simulink model "test"  (R2025a)
settings: Solver=VariableStepAuto  StartTime=0.0  StopTime=20  RelTol=1e-3
libraries: simulink_extras x2, aerolibanim x1, aerolibasang x1
settings Model: Creator=Ranvir  LastModifiedBy=Ranvir

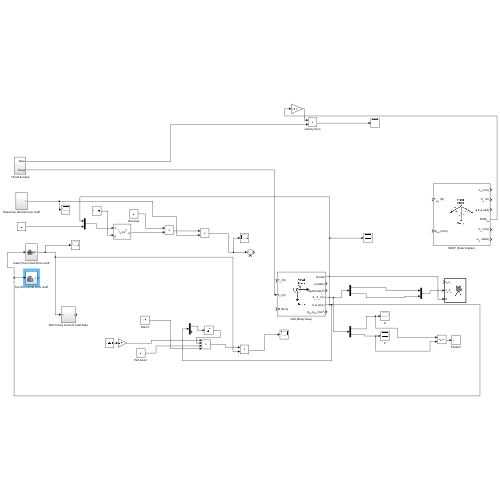
[thumbnail: Simulink's stored preview of the top-level diagram]
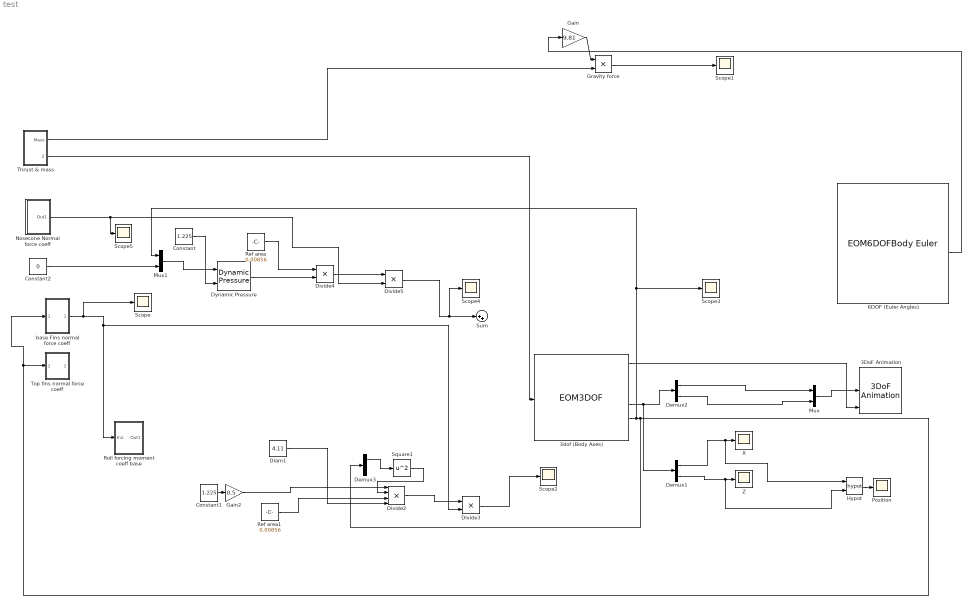
== system test ==
  3DoF Animation : aerolibanim/3DoF Animation  u1=[-25000 10000 -8000 2000 -15050 -3050]  u2=0.05  u3=1.0  u5=Fly alongside  u6=[1000 1000 1000]  u7=2  u8=on
  3dof (Body Axes) : EOM3DOF  v_ini=0  mass=36  Iyy=15
  6DOF (Euler Angles) : EOM6DOFBodyEuler  mass_0=36.51
  Constant : Constant  Value=1.225
  Constant1 : Constant  Value=1.225
  Constant2 : Constant  Value=0
  Demux1 : Demux  Outputs=2
  Demux2 : Demux  Outputs=2
  Demux3 : Demux  Outputs=2
  Diam1 : Constant  Value=4.11
  Divide2 : Product  Inputs=****
  Divide3 : Product  Inputs=**
  Divide4 : Product  Inputs=**
  Divide5 : Product  Inputs=**
  Dynamic Pressure : aerolibasang/Dynamic Pressure
  Gain : Gain  Gain=9.81
  Gain2 : Gain  Gain=0.5
  Gravity force : Product  Inputs=**
  Hypot : Math  Operator=hypot
  Mux : Mux  Inputs=2
  Mux1 : Mux  Inputs=2
  Nosecone Normal force coeff : Subsystem
  Position : Scope
      settings: ActiveDisplayYMinimum=-5509.2409156817193  ActiveDisplayYMaximum=105656.42411552551  DataLoggingVariableName=ScopeData7
  Ref area : Constant  Value=0.00856
  Ref area1 : Constant  Value=0.00856
  Roll forcing moment coeff base : Subsystem
  Scope{,1..5} (6 alike) : Scope
      Scope settings: ActiveDisplayYMinimum=9.6012949698591061  ActiveDisplayYMaximum=9.6019679428376143
      Scope1 settings: ActiveDisplayYMinimum=-90.814917446809943  ActiveDisplayYMaximum=480.58128367549506
      Scope2 settings: ActiveDisplayYMinimum=90.598933136696871  ActiveDisplayYMaximum=96.338960936146933  DataLoggingVariableName=ScopeData4
      Scope3 settings: ActiveDisplayYMinimum=318368.50157545973  ActiveDisplayYMaximum=399063.90685158595  DataLoggingVariableName=ScopeData5
      Scope4 settings: ActiveDisplayYMinimum=-1  ActiveDisplayYMaximum=1  DataLoggingVariableName=ScopeData8
      Scope5 settings: ActiveDisplayYMinimum=0.23621080058183891  ActiveDisplayYMaximum=0.2364376394256005  DataLoggingVariableName=ScopeData9
  Square1 : Math  Operator=square
  Sum : Sum  Inputs=|++
  Thrust & mass : Subsystem
  Top fins normal force coeff : Subsystem
  X : Scope
      settings: ActiveDisplayYMinimum=-6442.9252668406516  ActiveDisplayYMaximum=23566.686005062387  DataLoggingVariableName=ScopeData2
  Z : Scope
      settings: ActiveDisplayYMinimum=-39401.199186369508  ActiveDisplayYMaximum=178036.276331874  DataLoggingVariableName=ScopeData3
  base Fins normal force coeff : Subsystem
  wires:
  Divide5/1 -> Sum/1, Scope4/1
  Diam1/1 -> Divide2/4
  Square1/1 -> Divide2/2
  Divide4/1 -> Divide5/1
  Constant/1 -> Dynamic Pressure/2
  Mux1/1 -> Dynamic Pressure/1
  Divide2/1 -> Divide3/1
  Ref area1/1 -> Divide2/3
  Hypot/1 -> Position/1
  Demux2/1 -> Mux/1
  Demux2/2 -> Mux/2
  Demux1/1 -> Hypot/1, X/1
  Demux1/2 -> Hypot/2, Z/1
  Constant2/1 -> Mux1/2
  3dof (Body Axes)/1 -> 3DoF Animation/3
  Divide3/1 -> Scope2/1
  Dynamic Pressure/1 -> Divide4/2
  Nosecone Normal force coeff/1(Out1) -> Scope5/1, Divide5/2
  Ref area/1 -> Divide4/1
  Constant1/1 -> Gain2/1
  Thrust & mass/2(Thrust) -> 3dof (Body Axes)/2
  Mux/1 -> 3DoF Animation/2
  3dof (Body Axes)/4 -> Demux2/1, Demux1/1
  Demux3/1 -> Square1/1
  6DOF (Euler Angles)/4 -> Gain/1
  3dof (Body Axes)/5 -> base Fins normal force coeff/1(Velocity), Top fins normal force coeff/1(In1), Demux3/1, Scope3/1, Mux1/1
  Gain2/1 -> Divide2/1
  Thrust & mass/1(Mass) -> Gravity force/2
  Gravity force/1 -> Scope1/1
  base Fins normal force coeff/1(Out1) -> Scope/1, Divide3/2, Roll forcing moment coeff base/1(In1)
  Gain/1 -> Gravity force/1

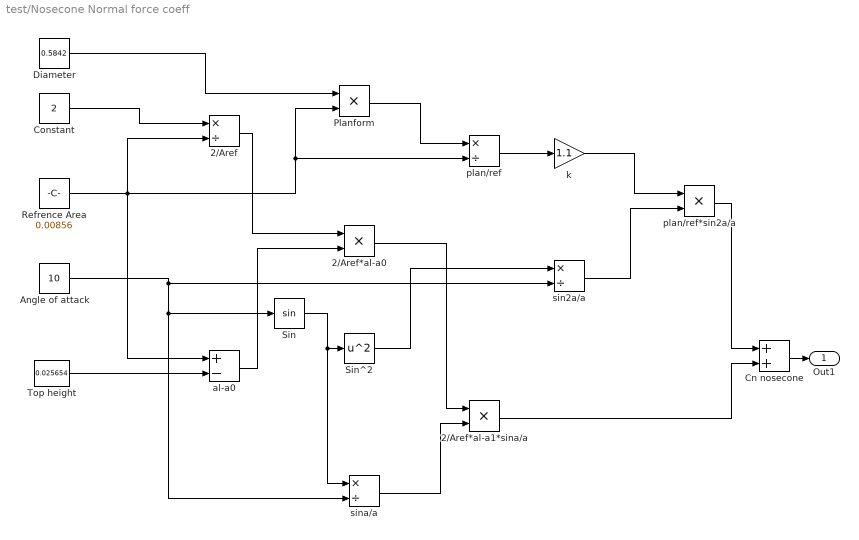
== system test/Nosecone Normal force coeff ==
  2/Aref : Product  Inputs=*/
  2/Aref*al-a0 : Product  Inputs=**
  2/Aref*al-a1*sina/a : Product  Inputs=**
  Angle of attack : Constant  Value=10
  Cn nosecone : Sum
  Constant : Constant  Value=2
  Diameter : Constant  Value=0.5842
  Planform : Product  Inputs=**
  Refrence Area : Constant  Value=0.00856
  Sin : Trigonometry
  Sin^2 : Math  Operator=square
  Top height : Constant  Value=0.025654
  al-a0 : Sum  Inputs=+-
  k : Gain  Gain=1.1
  plan/ref : Product  Inputs=*/
  plan/ref*sin2a/a : Product  Inputs=**
  sin2a/a : Product  Inputs=*/
  sina/a : Product  Inputs=*/
  Out1 : Outport
  wires:
  k/1 -> plan/ref*sin2a/a/1
  Refrence Area/1 -> plan/ref/2, Planform/2, 2/Aref/2, al-a0/1
  Sin^2/1 -> sin2a/a/1
  plan/ref/1 -> k/1
  Angle of attack/1 -> sin2a/a/2, Sin/1, sina/a/2
  al-a0/1 -> 2/Aref*al-a0/2
  2/Aref*al-a0/1 -> 2/Aref*al-a1*sina/a/1
  Sin/1 -> Sin^2/1, sina/a/1
  Diameter/1 -> Planform/1
  2/Aref/1 -> 2/Aref*al-a0/1
  Top height/1 -> al-a0/2
  sina/a/1 -> 2/Aref*al-a1*sina/a/2
  Constant/1 -> 2/Aref/1
  plan/ref*sin2a/a/1 -> Cn nosecone/1
  2/Aref*al-a1*sina/a/1 -> Cn nosecone/2
  Planform/1 -> plan/ref/1
  sin2a/a/1 -> plan/ref*sin2a/a/2
  Cn nosecone/1 -> Out1/1

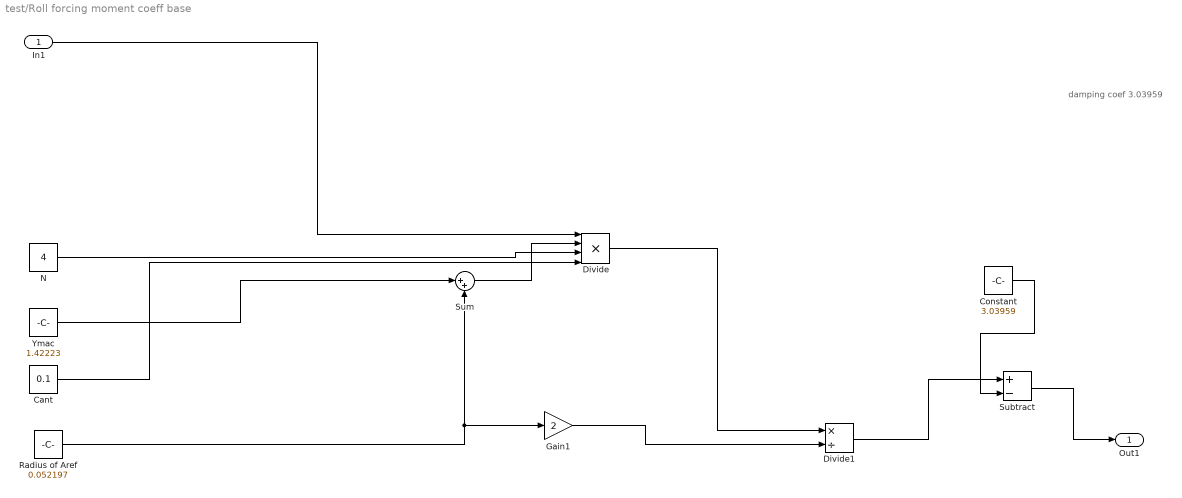
== system test/Roll forcing moment coeff base ==
  note: damping coef
      |  3.03959
  In1 : Inport
  Cant : Constant  Value=0.1
  Constant : Constant  Value=3.03959
  Divide : Product  Inputs=****
  Divide1 : Product  Inputs=*/
  Gain1 : Gain  Gain=2
  N : Constant  Value=4
  Radius of Aref : Constant  Value=0.052197
  Subtract : Sum  Inputs=+-
  Sum : Sum  Inputs=|++
  Ymac : Constant  Value=1.42223
  Out1 : Outport
  wires:
  Gain1/1 -> Divide1/2
  Divide/1 -> Divide1/1
  N/1 -> Divide/3
  Radius of Aref/1 -> Gain1/1, Sum/2
  Cant/1 -> Divide/4
  Ymac/1 -> Sum/1
  Sum/1 -> Divide/2
  In1/1 -> Divide/1
  Constant/1 -> Subtract/2
  Divide1/1 -> Subtract/1
  Subtract/1 -> Out1/1

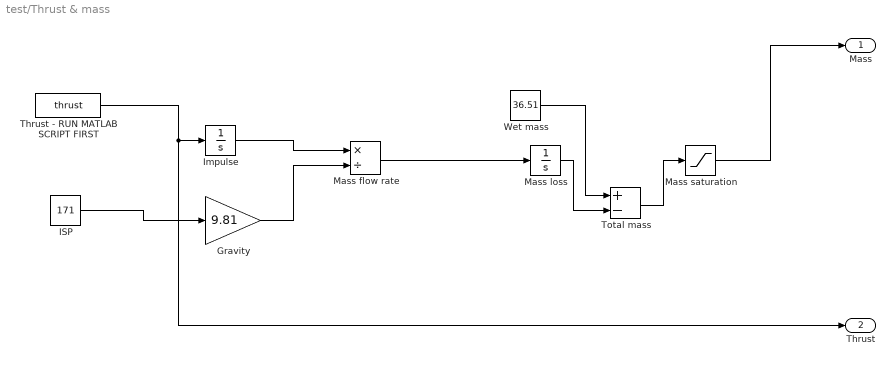
== system test/Thrust & mass ==
  Gravity : Gain  Gain=9.81
  ISP : Constant  Value=171
  Impulse : Integrator
  Mass flow rate : Product  Inputs=*/
  Mass loss : Integrator  UpperSaturationLimit=7  LowerSaturationLimit=0
  Mass saturation : Saturate  UpperLimit=36.51  LowerLimit=17.64
  Thrust - RUN MATLAB SCRIPT FIRST : FromWorkspace  VariableName=thrust  OutputAfterFinalValue=Setting to zero
  Total mass : Sum  Inputs=+-
  Wet mass : Constant  Value=36.51
  Mass : Outport
  Thrust : Outport  Port=2
  wires:
  Thrust - RUN MATLAB SCRIPT FIRST/1 -> Thrust/1, Impulse/1
  Total mass/1 -> Mass saturation/1
  Gravity/1 -> Mass flow rate/2
  Mass flow rate/1 -> Mass loss/1
  Wet mass/1 -> Total mass/1
  ISP/1 -> Gravity/1
  Impulse/1 -> Mass flow rate/1
  Mass loss/1 -> Total mass/2
  Mass saturation/1 -> Mass/1

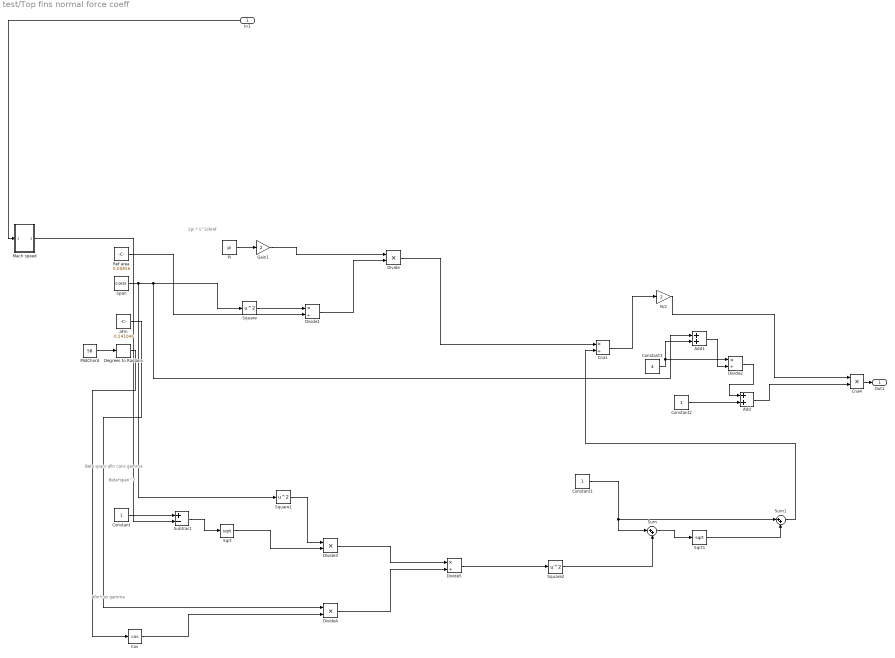
== system test/Top fins normal force coeff ==
  note: Afin*cos gamma
  note: Beta span/ afin cons gamma
  note: 2pi * s^2/Aref
  note: Beta*span^2
  In1 : Inport
  Add : Sum
  Add1 : Sum
  Cna1 : Product  Inputs=*/
  Cna4 : Product  Inputs=**
  Constant : Constant
  Constant1 : Constant
  Constant2 : Constant
  Constant3 : Constant  Value=4
  Cos : Trigonometry  Operator=cos
  Degrees to Radians : simulink_extras/Transformations/Degrees to Radians
  Divide : Product  Inputs=**
  Divide1 : Product  Inputs=*/
  Divide2 : Product  Inputs=*/
  Divide3 : Product  Inputs=**
  Divide4 : Product  Inputs=**
  Divide5 : Product  Inputs=*/
  Gain1 : Gain  Gain=2
  Mach speed : Subsystem
  MidChord : Constant  Value=58
  N/2 : Gain  Gain=2
  Pi : Constant  Value=pi  OutDataTypeStr=Inherit: Inherit via back propagation
  Ref area : Constant  Value=0.00856
  Span : Constant  Value=0.0635
  Sqrt : Sqrt
  Sqrt1 : Sqrt
  Square : Math  Operator=square
  Square1 : Math  Operator=square
  Square2 : Math  Operator=square
  Subtract : Sum  Inputs=+-
  Sum : Sum  Inputs=|++
  Sum1 : Sum  Inputs=|++
  aFin : Constant  Value=0.241046
  Out1 : Outport
  wires:
  aFin/1 -> Divide4/1
  Degrees to Radians/1 -> Cos/1
  MidChord/1 -> Degrees to Radians/1
  Sqrt1/1 -> Sum1/2
  In1/1 -> Mach speed/1(In1)
  Cna4/1 -> Out1/1
  Gain1/1 -> Divide/1
  Mach speed/1(Out1) -> Subtract/2
  Subtract/1 -> Sqrt/1
  Pi/1 -> Gain1/1
  Divide4/1 -> Divide5/2
  Add/1 -> Cna4/2
  Constant/1 -> Subtract/1
  Cna1/1 -> N/2/1
  Divide3/1 -> Divide5/1
  Divide2/1 -> Add/1
  N/2/1 -> Cna4/1
  Constant2/1 -> Add/2
  Span/1 -> Square1/1, Add1/1, Square/1
  Constant3/1 -> Add1/2, Divide2/1
  Divide1/1 -> Divide/2
  Ref area/1 -> Divide1/2
  Divide/1 -> Cna1/1
  Constant1/1 -> Sum1/1, Sum/1
  Sqrt/1 -> Divide3/2
  Square1/1 -> Divide3/1
  Sum1/1 -> Cna1/2
  Cos/1 -> Divide4/2
  Square2/1 -> Sum/2
  Divide5/1 -> Square2/1
  Square/1 -> Divide1/1
  Add1/1 -> Divide2/2
  Sum/1 -> Sqrt1/1

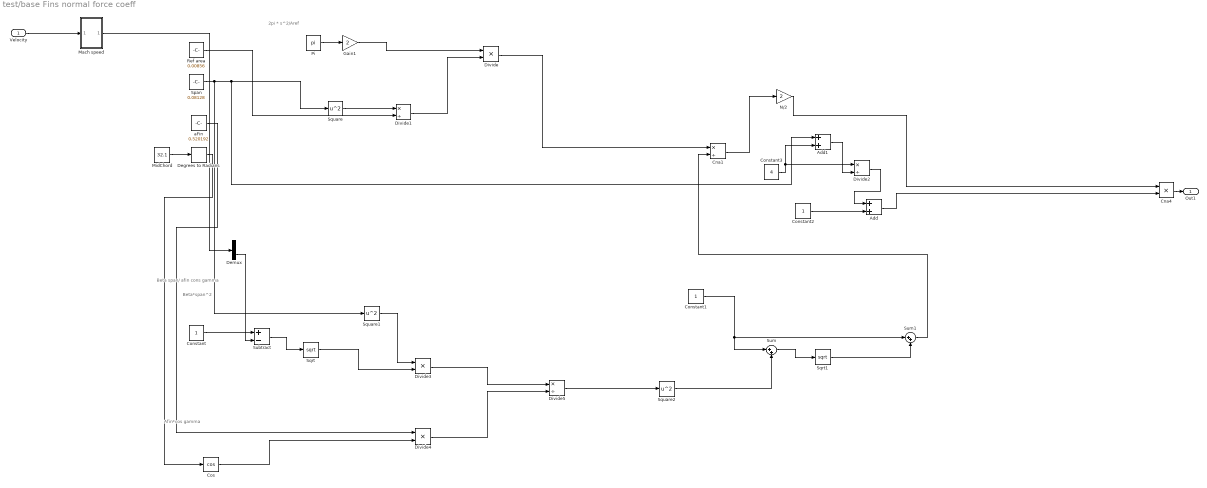
== system test/base Fins normal force coeff ==
  note: 2pi * s^2/Aref
  note: Beta span/ afin cons gamma
  note: Afin*cos gamma
  note: Beta*span^2
  Velocity : Inport
  Add : Sum
  Add1 : Sum
  Cna1 : Product  Inputs=*/
  Cna4 : Product  Inputs=**
  Constant : Constant
  Constant1 : Constant
  Constant2 : Constant
  Constant3 : Constant  Value=4
  Cos : Trigonometry  Operator=cos
  Degrees to Radians : simulink_extras/Transformations/Degrees to Radians
  Demux : Demux  Outputs=2
  Divide : Product  Inputs=**
  Divide1 : Product  Inputs=*/
  Divide2 : Product  Inputs=*/
  Divide3 : Product  Inputs=**
  Divide4 : Product  Inputs=**
  Divide5 : Product  Inputs=*/
  Gain1 : Gain  Gain=2
  Mach speed : Subsystem
  MidChord : Constant  Value=32.1
  N/2 : Gain  Gain=2
  Pi : Constant  Value=pi  OutDataTypeStr=Inherit: Inherit via back propagation
  Ref area : Constant  Value=0.00856
  Span : Constant  Value=0.08128
  Sqrt : Sqrt
  Sqrt1 : Sqrt
  Square : Math  Operator=square
  Square1 : Math  Operator=square
  Square2 : Math  Operator=square
  Subtract : Sum  Inputs=+-
  Sum : Sum  Inputs=|++
  Sum1 : Sum  Inputs=|++
  aFin : Constant  Value=0.520192
  Out1 : Outport
  wires:
  Constant1/1 -> Sum1/1, Sum/1
  Span/1 -> Square1/1, Add1/1, Square/1
  Gain1/1 -> Divide/1
  Divide/1 -> Cna1/1
  Ref area/1 -> Divide1/2
  Constant2/1 -> Add/2
  Add/1 -> Cna4/2
  Add1/1 -> Divide2/2
  Sqrt/1 -> Divide3/2
  Divide2/1 -> Add/1
  Constant3/1 -> Add1/2, Divide2/1
  Constant/1 -> Subtract/1
  Divide4/1 -> Divide5/2
  N/2/1 -> Cna4/1
  Pi/1 -> Gain1/1
  aFin/1 -> Divide4/1
  Divide3/1 -> Divide5/1
  MidChord/1 -> Degrees to Radians/1
  Subtract/1 -> Sqrt/1
  Velocity/1 -> Mach speed/1(In1)
  Sqrt1/1 -> Sum1/2
  Divide5/1 -> Square2/1
  Square1/1 -> Divide3/1
  Square2/1 -> Sum/2
  Degrees to Radians/1 -> Cos/1
  Cna1/1 -> N/2/1
  Square/1 -> Divide1/1
  Mach speed/1(Out1) -> Demux/1
  Cos/1 -> Divide4/2
  Sum/1 -> Sqrt1/1
  Divide1/1 -> Divide/2
  Sum1/1 -> Cna1/2
  Cna4/1 -> Out1/1
  Demux/2 -> Subtract/2

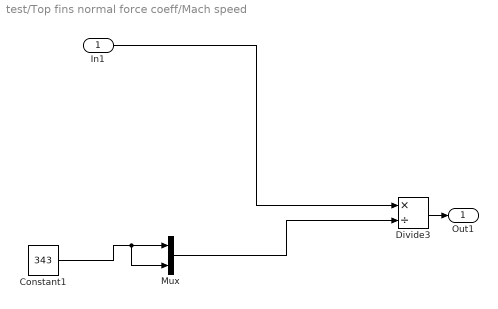
== system test/Top fins normal force coeff/Mach speed ==
  In1 : Inport
  Constant1 : Constant  Value=343
  Divide3 : Product  Inputs=*/
  Mux : Mux  Inputs=2
  Out1 : Outport
  wires:
  Mux/1 -> Divide3/2
  Constant1/1 -> Mux/2, Mux/1
  In1/1 -> Divide3/1
  Divide3/1 -> Out1/1

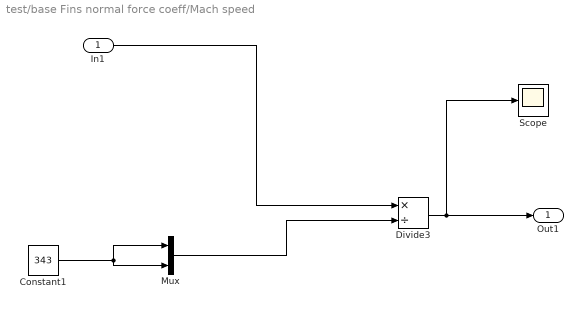
== system test/base Fins normal force coeff/Mach speed ==
  In1 : Inport
  Constant1 : Constant  Value=343
  Divide3 : Product  Inputs=*/
  Mux : Mux  Inputs=2
  Scope : Scope
      settings: ActiveDisplayYMinimum=-5.3370529359830341  ActiveDisplayYMaximum=7.5551253883729084  DataLoggingVariableName=ScopeData6
  Out1 : Outport
  wires:
  Mux/1 -> Divide3/2
  Constant1/1 -> Mux/1, Mux/2
  In1/1 -> Divide3/1
  Divide3/1 -> Scope/1, Out1/1
